simulink model "FinalMMDmodel"  (R2024b)
settings: Solver=VariableStepAuto  StartTime=0.0  StopTime=30  RelTol=1e-3
values from neighbouring files (symbols this model uses):
  combinedmass = m1+m2    (= 305)    [AllModels.m]
  g = 9.81    [AllModels.m]    (also in workspace_variables.mat)
  K_lqr = lqr(A, B, Q, R)    [AllModels.m]    (also in workspace_variables.mat = [5.47722557505 58.0638895637 8.67973677662 104.310428086])
  l = 2.5    [AllModels.m]    (also in workspace_variables.mat)
  m1 = 250    [AllModels.m]    (also in workspace_variables.mat)
  m2 = 55    [AllModels.m]    (also in workspace_variables.mat)
libraries: slpidlib x2
settings Model: Creator=Hadi  LastModifiedBy=Lenovo

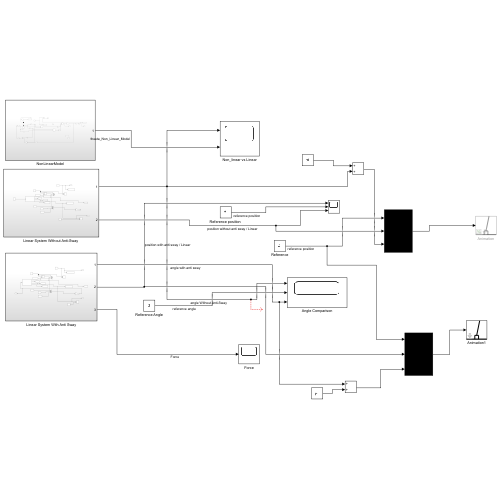
[thumbnail: Simulink's stored preview of the top-level diagram]
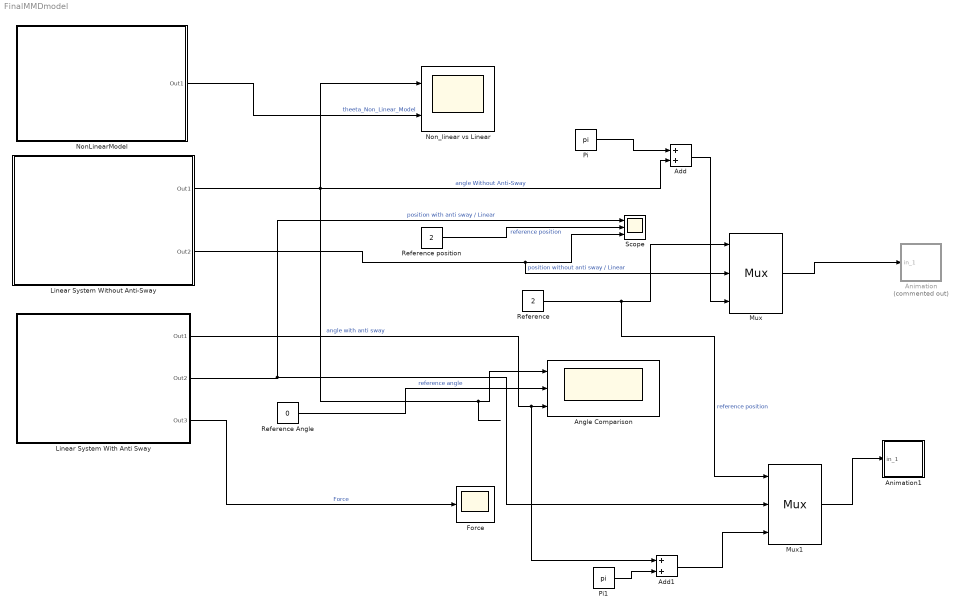
== system FinalMMDmodel ==
  Add : Sum
  Add1 : Sum
  Angle Comparison : Scope  NumInputPorts=3
  Animation : Subsystem  Commented=on  mask(Pendulum plot){RefBlock=Reference}
      mask prompts: RefBlock "DC reference signal block name:"
      mask help: Pendulum plot
      mask Help: Pendulum animation function using Handle graphics.
      mask Display: plot([-10 10],[0 0],[-2 -2 2 2],[0 1 1 0],[0 3],[1 5])
  Animation1 : Subsystem  mask(Pendulum plot){RefBlock=Reference}
      mask prompts: RefBlock "DC reference signal block name:"
      mask help: Pendulum plot
      mask Help: Pendulum animation function using Handle graphics.
      mask Display: plot([-10 10],[0 0],[-2 -2 2 2],[0 1 1 0],[0 3],[1 5])
  Force : Scope
  Linear System With Anti Sway : Subsystem
  "Linear System Without Anti-Sway " : Subsystem
  Mux : Mux  Inputs=3
  Mux1 : Mux  Inputs=3
  NonLinearModel : Subsystem
  Non_linear vs Linear : Scope  NumInputPorts=2
  Pi : Constant  Value=pi  OutDataTypeStr=Inherit: Inherit via back propagation
  Pi1 : Constant  Value=pi  OutDataTypeStr=Inherit: Inherit via back propagation
  Reference : Constant  Value=2
  Reference Angle : Constant  Value=0
  "Reference position " : Constant  Value=2
  Scope : Scope  NumInputPorts=3
  wires:
  "Linear System Without Anti-Sway "/1(Out1) -> Add/2, Non_linear vs Linear/1, Angle Comparison/1  "angle Without Anti-Sway"
  Linear System With Anti Sway/1(Out1) -> Add1/1, Angle Comparison/3  "angle with anti sway"
  Reference Angle/1 -> Angle Comparison/2  "reference angle"
  "Linear System Without Anti-Sway "/2(Out2) -> Mux/2, Scope/3  "position without anti sway / Linear"
  Linear System With Anti Sway/2(Out2) -> Mux1/2, Scope/1  "position with anti sway / Linear"
  Reference/1 -> Mux1/1, Mux/1  "reference position"
  NonLinearModel/1(Out1) -> Non_linear vs Linear/2  "theeta_Non_Linear_Model"
  Linear System With Anti Sway/3(Out3) -> Force/1  "Force"
  Mux/1 -> Animation/1(in_1)
  Pi/1 -> Add/1
  Add/1 -> Mux/3
  Mux1/1 -> Animation1/1(in_1)
  "Reference position "/1 -> Scope/2  "reference position"
  Pi1/1 -> Add1/2
  Add1/1 -> Mux1/3

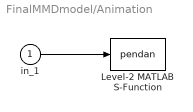
== system FinalMMDmodel/Animation ==
  in_1 : Inport
  Level-2 MATLAB S-Function : M-S-Function  FunctionName=pendan  Parameters=RefBlock
  wires:
  in_1/1 -> Level-2 MATLAB S-Function/1

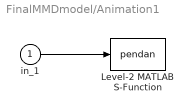
== system FinalMMDmodel/Animation1 ==
  in_1 : Inport
  Level-2 MATLAB S-Function : M-S-Function  FunctionName=pendan  Parameters=RefBlock
  wires:
  in_1/1 -> Level-2 MATLAB S-Function/1

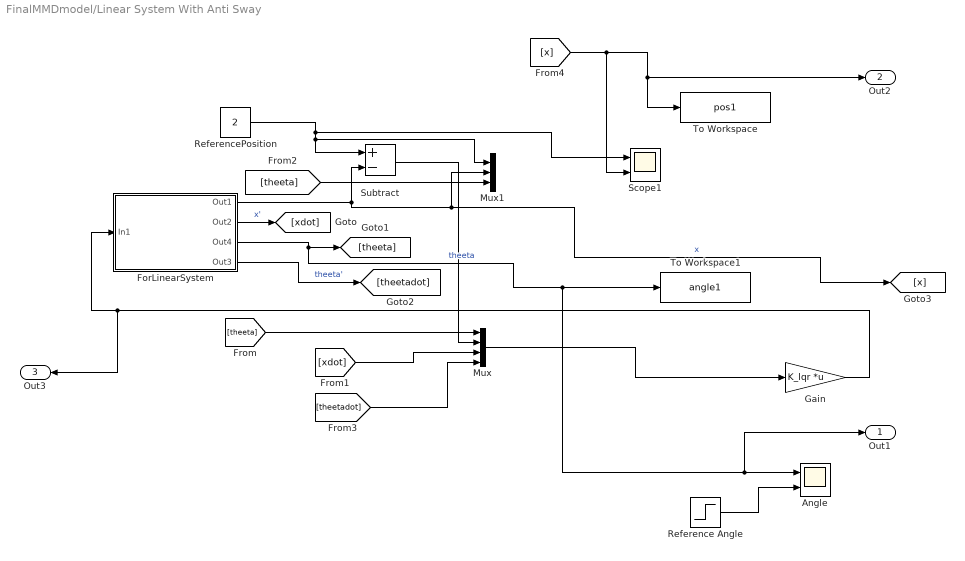
== system FinalMMDmodel/Linear System With Anti Sway ==
  Angle : Scope  NumInputPorts=2
  ForLinearSystem : Subsystem
  Gain : Gain  Gain=K_lqr  Multiplication=Matrix(K*u)
  Mux : Mux
  Mux1 : Mux  Inputs=3
  Reference Angle : Step  After=0  SampleTime=0
  ReferencePosition : Constant  Value=2
  Scope1 : Scope  NumInputPorts=2
  Subtract : Sum  Inputs=+-
  To Workspace : ToWorkspace  VariableName=pos1  SaveFormat=Timeseries  SampleTime=-1
  To Workspace1 : ToWorkspace  VariableName=angle1  SaveFormat=Timeseries  SampleTime=-1
  Out1 : Outport
  Out2 : Outport  Port=2
  Out3 : Outport  Port=3
  wires:
  Mux/1 -> Gain/1
  ForLinearSystem/3(Out4) -> Out1/1, Angle/1, To Workspace1/1, [theeta]  "theeta"
  ForLinearSystem/2(Out2) -> [xdot]  "x'"
  [theeta] -> Mux1/3
  Subtract/1 -> Mux/2
  ForLinearSystem/1(Out1) -> Mux1/2, [x], Subtract/2  "x"
  Reference Angle/1 -> Angle/2
  ReferencePosition/1 -> Scope1/1, Mux1/1, Subtract/1
  [x] -> Out2/1, To Workspace/1, Scope1/2
  ForLinearSystem/4(Out3) -> [theetadot]  "theeta'"
  [theetadot] -> Mux/4
  Gain/1 -> Out3/1, ForLinearSystem/1(In1)
  [theeta] -> Mux/1
  [xdot] -> Mux/3

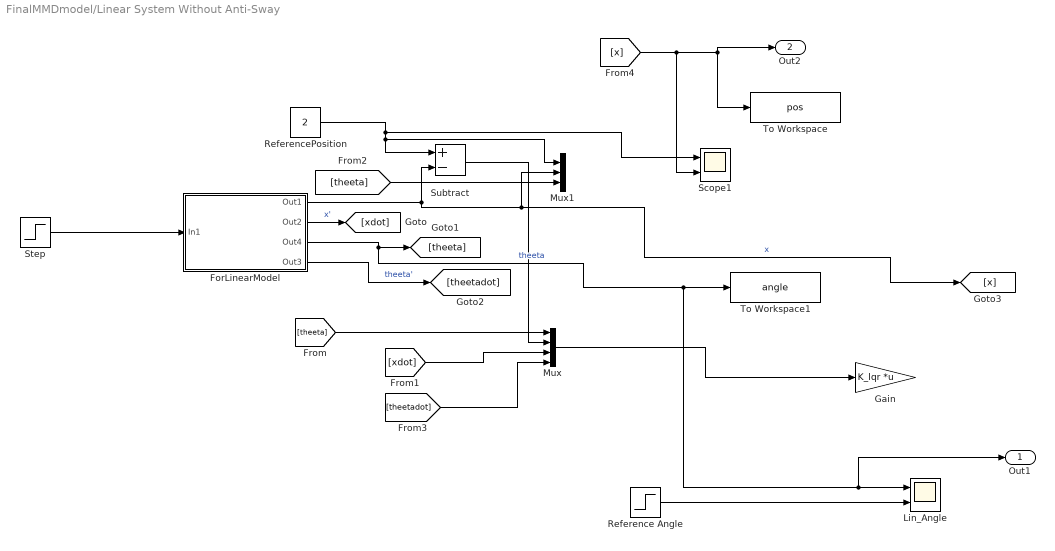
== system FinalMMDmodel/Linear System Without Anti-Sway  ==
  ForLinearModel : Subsystem
  Gain : Gain  Gain=K_lqr  Multiplication=Matrix(K*u)
  Lin_Angle : Scope  NumInputPorts=2
  Mux : Mux
  Mux1 : Mux  Inputs=3
  Reference Angle : Step  After=0  SampleTime=0
  ReferencePosition : Constant  Value=2
  Scope1 : Scope  NumInputPorts=2
  Step : Step  Time=0  After=200  SampleTime=0
  Subtract : Sum  Inputs=+-
  To Workspace : ToWorkspace  VariableName=pos  SaveFormat=Timeseries  SampleTime=-1
  To Workspace1 : ToWorkspace  VariableName=angle  SaveFormat=Timeseries  SampleTime=-1
  Out1 : Outport
  Out2 : Outport  Port=2
  wires:
  [theetadot] -> Mux/4
  [xdot] -> Mux/3
  ForLinearModel/1(Out1) -> Mux1/2, [x], Subtract/2  "x"
  [theeta] -> Mux/1
  ForLinearModel/4(Out3) -> [theetadot]  "theeta'"
  [x] -> To Workspace/1, Out2/1, Scope1/2
  Reference Angle/1 -> Lin_Angle/2
  Step/1 -> ForLinearModel/1(In1)
  Subtract/1 -> Mux/2
  ForLinearModel/2(Out2) -> [xdot]  "x'"
  ReferencePosition/1 -> Scope1/1, Mux1/1, Subtract/1
  ForLinearModel/3(Out4) -> Out1/1, Lin_Angle/1, To Workspace1/1, [theeta]  "theeta"
  Mux/1 -> Gain/1
  [theeta] -> Mux1/3

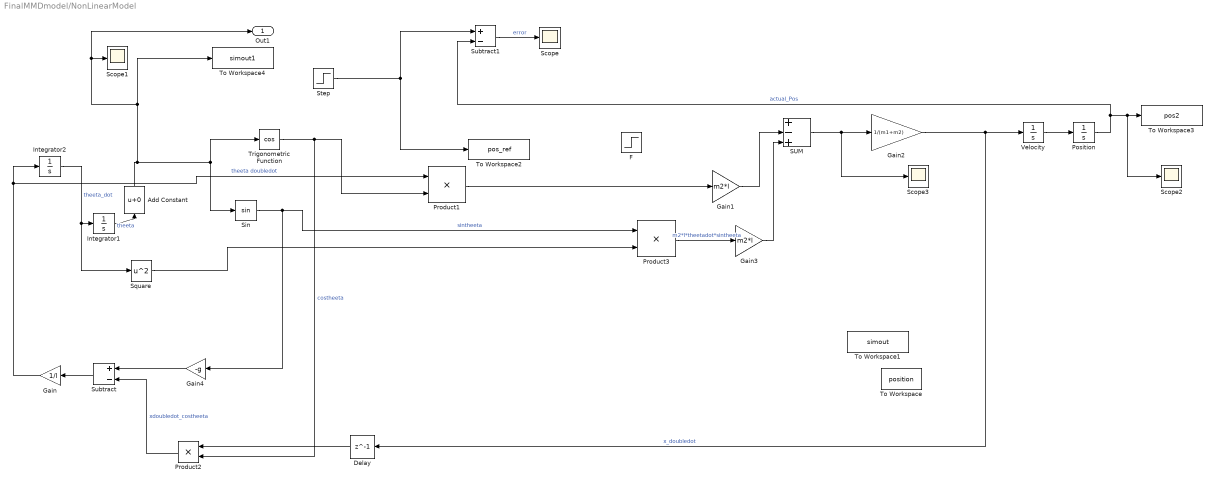
== system FinalMMDmodel/NonLinearModel ==
  Add Constant : Bias  SaturateOnIntegerOverflow=off
  Delay : Delay  DelayLength=1
  F : Step  Time=0  After=200  SampleTime=0
  Gain : Gain  Gain=1/l
  Gain1 : Gain  Gain=m2*l
  Gain2 : Gain  Gain=1/(m1+m2)
  Gain3 : Gain  Gain=m2*l
  Gain4 : Gain  Gain=-g
  Integrator1 : Integrator
  Integrator2 : Integrator
  Position : Integrator
  Product1 : Product
  Product2 : Product
  Product3 : Product
  SUM : Sum  Inputs=+-+
  Scope{,1..3} (4 alike) : Scope
  Sin : Trigonometry
  Square : Math  Operator=square
  Step : Step  After=2  SampleTime=0
  Subtract : Sum  Inputs=+-
  Subtract1 : Sum  Inputs=+-
  To Workspace : ToWorkspace  VariableName=position  SaveFormat=Timeseries  SampleTime=-1
  To Workspace1 : ToWorkspace  VariableName=simout  SaveFormat=Timeseries  SampleTime=-1
  To Workspace2 : ToWorkspace  VariableName=pos_ref  SaveFormat=Timeseries  SampleTime=-1
  To Workspace3 : ToWorkspace  VariableName=pos2  SaveFormat=Timeseries  SampleTime=-1
  To Workspace4 : ToWorkspace  VariableName=simout1  SaveFormat=Timeseries  SampleTime=-1
  Trigonometric Function : Trigonometry  Operator=cos
  Velocity : Integrator
  Out1 : Outport
  wires:
  Integrator2/1 -> Square/1, Integrator1/1  "theeta_dot"
  Trigonometric Function/1 -> Product2/2, Product1/2  "costheeta"
  Product3/1 -> Gain3/1  "m2*l*theetadot*sintheeta"
  Sin/1 -> Gain4/1, Product3/1  "sintheeta"
  Velocity/1 -> Position/1
  Integrator1/1 -> Add Constant/1  "theeta"
  Subtract1/1 -> Scope/1  "error"
  Product2/1 -> Subtract/2  "xdoubledot_costheeta"
  SUM/1 -> Scope3/1, Gain2/1
  Position/1 -> Scope2/1, To Workspace3/1, Subtract1/2  "actual_Pos"
  Gain4/1 -> Subtract/1
  Delay/1 -> Product2/1
  Gain/1 -> Integrator2/1, Product1/1  "theeta doubledot"
  Square/1 -> Product3/2
  Product1/1 -> Gain1/1
  Gain2/1 -> Delay/1, Velocity/1  "x_doubledot"
  Step/1 -> To Workspace2/1, Subtract1/1
  Gain1/1 -> SUM/2
  Subtract/1 -> Gain/1
  Gain3/1 -> SUM/3
  Add Constant/1 -> Sin/1, Trigonometric Function/1, Out1/1, Scope1/1, To Workspace4/1

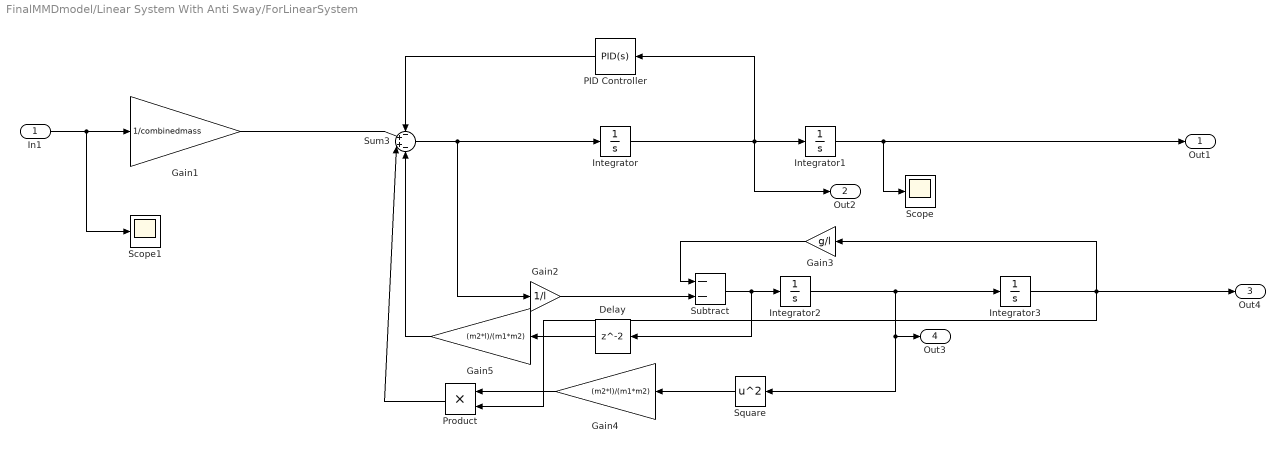
== system FinalMMDmodel/Linear System With Anti Sway/ForLinearSystem ==
  In1 : Inport
  Delay : Delay
  Gain1 : Gain  Gain=1/combinedmass
  Gain2 : Gain  Gain=1/l
  Gain3 : Gain  Gain=g/l
  Gain4 : Gain  Gain=(m2*l)/(m1*m2)
  Gain5 : Gain  Gain=(m2*l)/(m1*m2)
  Integrator{,1..3} (4 alike) : Integrator
  PID Controller : slpidlib/PID Controller  Controller=PID  Form=Parallel  TimeDomain=Continuous-time  UseExternalTs=off  SampleTime=-1  IntegratorMethod=Forward Euler  FilterMethod=Forward Euler  ControllerParametersSource=internal  P=0.4  I=0  UseKiTs=off  D=1  UseExternalDerivativeSource=off  N=100  UseFilter=on  TunerSelectOption=Transfer Function Based (PID Tuner App)  InitialConditionSource=internal  InitialConditionForIntegrator=0  InitialConditionForFilter=0  DifferentiatorICPrevScaledInput=0  ExternalReset=none  TrackingMode=off  Kt=1  LimitOutput=off  SatLimitsSource=internal  UpperSaturationLimit=inf  LowerSaturationLimit=-inf  LinearizeAsGain=on  AntiWindupMode=none  Kb=1  LimitIntegrator=off  UpperIntegratorSaturationLimit=inf  LowerIntegratorSaturationLimit=-inf  POutMin=[]  POutMax=[]  IOutMin=[]  IOutMax=[]  DOutMin=[]  DOutMax=[]  NOutMin=[]  NOutMax=[]  SumOutMin=[]  SumOutMax=[]  SaturationOutMin=[]  SaturationOutMax=[]  PParamMin=[]  PParamMax=[]  IParamMin=[]  IParamMax=[]  DParamMin=[]  DParamMax=[]  NParamMin=[]  NParamMax=[]  KbParamMin=[]  KbParamMax=[]  KtParamMin=[]  KtParamMax=[]  KbOutMin=[]  KbOutMax=[]  KtOutMin=[]  KtOutMax=[]  IntegratorOutMin=[]  IntegratorOutMax=[]  FilterOutMin=[]  FilterOutMax=[]  SumI1OutMin=[]  SumI1OutMax=[]  SumI2OutMin=[]  SumI2OutMax=[]  SumI3OutMin=[]  SumI3OutMax=[]  SumI4OutMin=[]  SumI4OutMax=[]  SumDOutMin=[]  SumDOutMax=[]  DifferentiatorOutMin=[]  DifferentiatorOutMax=[]  FilterDiffOutCoefMin=[]  FilterDiffOutCoefMax=[]  ReciprocalOutMin=[]  ReciprocalOutMax=[]  SumDenOutMin=[]  SumDenOutMax=[]  SumNumOutMin=[]  SumNumOutMax=[]  DivideOutMin=[]  DivideOutMax=[]  UdiffTsProdOutMin=[]  UdiffTsProdOutMax=[]  NTsProdOutMin=[]  NTsProdOutMax=[]  UintegralTsProdOutMin=[]  UintegralTsProdOutMax=[]  UngainTsProdOutMin=[]  UngainTsProdOutMax=[]  ClampingZeroOutDataTypeStr=Inherit: Inherit via back propagation  ClampingZeroOutMin=[]  ClampingZeroOutMax=[]  FilterDenConstantOutDataTypeStr=Inherit: Inherit via back propagation  FilterDenConstantOutMin=[]  FilterDenConstantOutMax=[]  PCopyOutDataTypeStr=Inherit: Inherit via back propagation  PCopyOutMin=[]  PCopyOutMax=[]  NCopyOutDataTypeStr=Inherit: Inherit via back propagation  NCopyOutMin=[]  NCopyOutMax=[]  IntegratorContinuousStateAttributes=''  IntegratorStateMustResolveToSignalObject=off  IntegratorRTWStateStorageClass=Auto  FilterContinuousStateAttributes=''  FilterStateMustResolveToSignalObject=off  FilterRTWStateStorageClass=Auto  ParallelPVariant=InternalParameters  IdealPVariant=Disabled  IVariant=InternalParameters  DVariant=InternalParameters  IntegratorVariant=Continuous  SatVariant=Disabled  AWVariant=Passthrough  PCopyVariant=Disabled  TRVariant=Disabled  FdbkBlocksVariant=Forward  IdealPFdbkVariant=Disabled  SatFdbkVariant=Disabled  DerivativeFilterVariant=ContFilter  NVariant=InternalParameters  NCopyVariant=Disabled  FilterICVariant=InternalICsFilter  IntegratorICVariant=InternalICs  ExternalResetVariant=Disabled  TRSumVariant=Passthrough  SumFdbkVariant=Disabled  SumVariant=Sum_PID  TsampFilterVariant=InternalTs  TsampNgainVariant=Passthrough  TsampIntegralVariant=Disabled_SignalSpec  ExternalSaturationOutDataTypeStr=Inherit: Same as second input  DerivativeSourceVariant=ErrorSignal  PreIntVariant=InternalPreInt
  Product : Product
  Scope : Scope
  Scope1 : Scope
  Square : Math  Operator=square
  Subtract : Sum  Inputs=--
  Sum3 : Sum  Inputs=-++-
  Out1 : Outport
  Out2 : Outport  Port=2
  Out4 : Outport  Port=3
  Out3 : Outport  Port=4
  wires:
  Gain1/1 -> Sum3/2
  Gain3/1 -> Subtract/1
  Integrator3/1 -> Product/2, Out4/1, Gain3/1
  Sum3/1 -> Gain2/1, Integrator/1
  Integrator2/1 -> Square/1, Out3/1, Integrator3/1
  Integrator1/1 -> Out1/1, Scope/1
  PID Controller/1 -> Sum3/1
  Gain2/1 -> Subtract/2
  Gain4/1 -> Product/1
  In1/1 -> Scope1/1, Gain1/1
  Product/1 -> Sum3/3
  Integrator/1 -> PID Controller/1, Out2/1, Integrator1/1
  Subtract/1 -> Delay/1, Integrator2/1
  Square/1 -> Gain4/1
  Gain5/1 -> Sum3/4
  Delay/1 -> Gain5/1

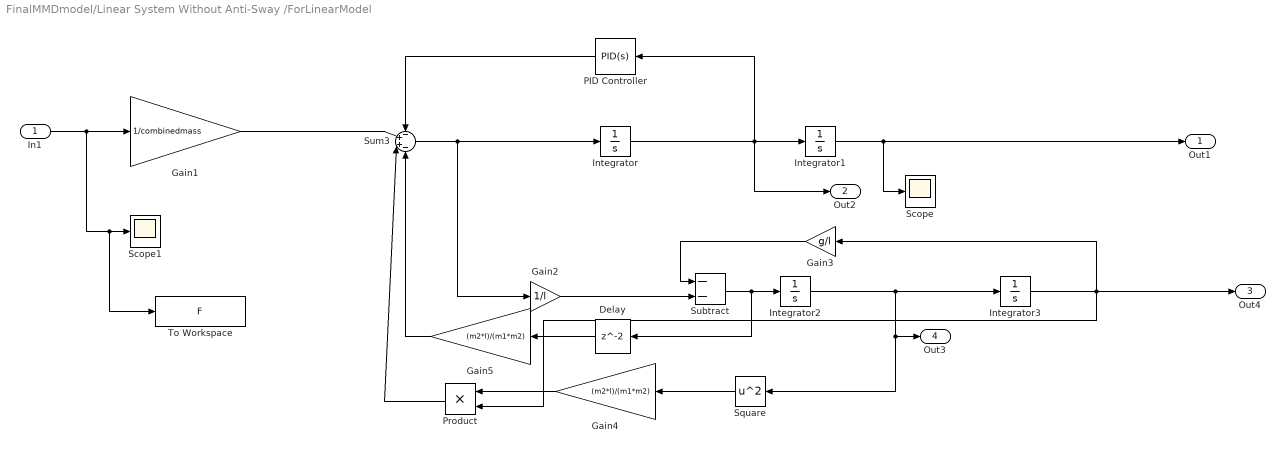
== system FinalMMDmodel/Linear System Without Anti-Sway /ForLinearModel ==
  In1 : Inport
  Delay : Delay
  Gain1 : Gain  Gain=1/combinedmass
  Gain2 : Gain  Gain=1/l
  Gain3 : Gain  Gain=g/l
  Gain4 : Gain  Gain=(m2*l)/(m1*m2)
  Gain5 : Gain  Gain=(m2*l)/(m1*m2)
  Integrator{,1..3} (4 alike) : Integrator
  PID Controller : slpidlib/PID Controller  Controller=PID  Form=Parallel  TimeDomain=Continuous-time  UseExternalTs=off  SampleTime=-1  IntegratorMethod=Forward Euler  FilterMethod=Forward Euler  ControllerParametersSource=internal  P=0.4  I=0  UseKiTs=off  D=1  UseExternalDerivativeSource=off  N=100  UseFilter=on  TunerSelectOption=Transfer Function Based (PID Tuner App)  InitialConditionSource=internal  InitialConditionForIntegrator=0  InitialConditionForFilter=0  DifferentiatorICPrevScaledInput=0  ExternalReset=none  TrackingMode=off  Kt=1  LimitOutput=off  SatLimitsSource=internal  UpperSaturationLimit=inf  LowerSaturationLimit=-inf  LinearizeAsGain=on  AntiWindupMode=none  Kb=1  LimitIntegrator=off  UpperIntegratorSaturationLimit=inf  LowerIntegratorSaturationLimit=-inf  POutMin=[]  POutMax=[]  IOutMin=[]  IOutMax=[]  DOutMin=[]  DOutMax=[]  NOutMin=[]  NOutMax=[]  SumOutMin=[]  SumOutMax=[]  SaturationOutMin=[]  SaturationOutMax=[]  PParamMin=[]  PParamMax=[]  IParamMin=[]  IParamMax=[]  DParamMin=[]  DParamMax=[]  NParamMin=[]  NParamMax=[]  KbParamMin=[]  KbParamMax=[]  KtParamMin=[]  KtParamMax=[]  KbOutMin=[]  KbOutMax=[]  KtOutMin=[]  KtOutMax=[]  IntegratorOutMin=[]  IntegratorOutMax=[]  FilterOutMin=[]  FilterOutMax=[]  SumI1OutMin=[]  SumI1OutMax=[]  SumI2OutMin=[]  SumI2OutMax=[]  SumI3OutMin=[]  SumI3OutMax=[]  SumI4OutMin=[]  SumI4OutMax=[]  SumDOutMin=[]  SumDOutMax=[]  DifferentiatorOutMin=[]  DifferentiatorOutMax=[]  FilterDiffOutCoefMin=[]  FilterDiffOutCoefMax=[]  ReciprocalOutMin=[]  ReciprocalOutMax=[]  SumDenOutMin=[]  SumDenOutMax=[]  SumNumOutMin=[]  SumNumOutMax=[]  DivideOutMin=[]  DivideOutMax=[]  UdiffTsProdOutMin=[]  UdiffTsProdOutMax=[]  NTsProdOutMin=[]  NTsProdOutMax=[]  UintegralTsProdOutMin=[]  UintegralTsProdOutMax=[]  UngainTsProdOutMin=[]  UngainTsProdOutMax=[]  ClampingZeroOutDataTypeStr=Inherit: Inherit via back propagation  ClampingZeroOutMin=[]  ClampingZeroOutMax=[]  FilterDenConstantOutDataTypeStr=Inherit: Inherit via back propagation  FilterDenConstantOutMin=[]  FilterDenConstantOutMax=[]  PCopyOutDataTypeStr=Inherit: Inherit via back propagation  PCopyOutMin=[]  PCopyOutMax=[]  NCopyOutDataTypeStr=Inherit: Inherit via back propagation  NCopyOutMin=[]  NCopyOutMax=[]  IntegratorContinuousStateAttributes=''  IntegratorStateMustResolveToSignalObject=off  IntegratorRTWStateStorageClass=Auto  FilterContinuousStateAttributes=''  FilterStateMustResolveToSignalObject=off  FilterRTWStateStorageClass=Auto  ParallelPVariant=InternalParameters  IdealPVariant=Disabled  IVariant=InternalParameters  DVariant=InternalParameters  IntegratorVariant=Continuous  SatVariant=Disabled  AWVariant=Passthrough  PCopyVariant=Disabled  TRVariant=Disabled  FdbkBlocksVariant=Forward  IdealPFdbkVariant=Disabled  SatFdbkVariant=Disabled  DerivativeFilterVariant=ContFilter  NVariant=InternalParameters  NCopyVariant=Disabled  FilterICVariant=InternalICsFilter  IntegratorICVariant=InternalICs  ExternalResetVariant=Disabled  TRSumVariant=Passthrough  SumFdbkVariant=Disabled  SumVariant=Sum_PID  TsampFilterVariant=InternalTs  TsampNgainVariant=Passthrough  TsampIntegralVariant=Disabled_SignalSpec  ExternalSaturationOutDataTypeStr=Inherit: Same as second input  DerivativeSourceVariant=ErrorSignal  PreIntVariant=InternalPreInt
  Product : Product
  Scope : Scope
  Scope1 : Scope
  Square : Math  Operator=square
  Subtract : Sum  Inputs=--
  Sum3 : Sum  Inputs=-++-
  To Workspace : ToWorkspace  VariableName=F  SaveFormat=Timeseries  SampleTime=-1
  Out1 : Outport
  Out2 : Outport  Port=2
  Out4 : Outport  Port=3
  Out3 : Outport  Port=4
  wires:
  Gain1/1 -> Sum3/2
  Gain3/1 -> Subtract/1
  Integrator3/1 -> Product/2, Out4/1, Gain3/1
  Sum3/1 -> Gain2/1, Integrator/1
  Integrator2/1 -> Square/1, Out3/1, Integrator3/1
  Integrator1/1 -> Out1/1, Scope/1
  PID Controller/1 -> Sum3/1
  Gain2/1 -> Subtract/2
  Gain4/1 -> Product/1
  In1/1 -> To Workspace/1, Scope1/1, Gain1/1
  Product/1 -> Sum3/3
  Integrator/1 -> PID Controller/1, Out2/1, Integrator1/1
  Subtract/1 -> Delay/1, Integrator2/1
  Square/1 -> Gain4/1
  Gain5/1 -> Sum3/4
  Delay/1 -> Gain5/1
